simulink model "Copy_of_RoboCarModel"  (R2023a)
settings: Solver=VariableStepAuto  StartTime=0.0  StopTime=10.0  RelTol=1e-3
settings Model: Creator=Franz  LastModifiedBy=Franz

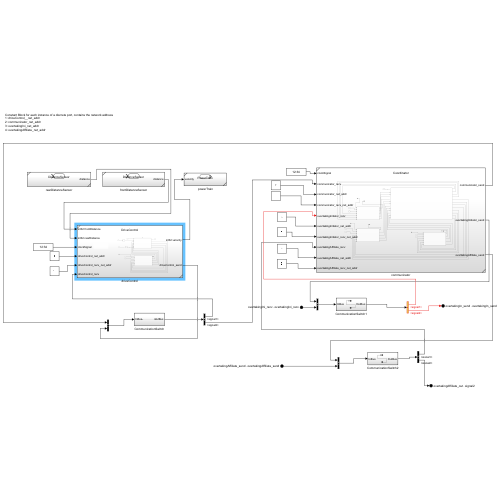
[thumbnail: Simulink's stored preview of the top-level diagram]
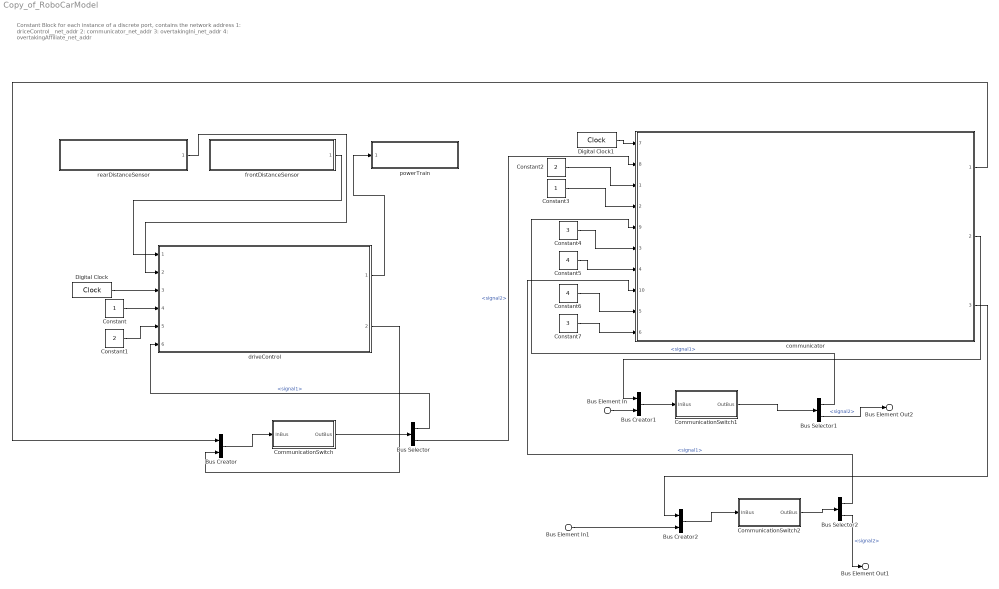
== system Copy_of_RoboCarModel ==
  note: Constant Block for each instance of a discrete port, contains the network address
      | 1: driceControl__net_addr
      | 2: communicator_net_addr
      | 3: overtakingIni_net_addr
      | 4: overtakingAffiliate_net_addr
  Bus Element In : Inport  PortName=overtakingIni_recv  Element=overtakingIni_recv
  Bus Element In1 : Inport  Port=2  PortName=overtakingAffiliate_send  Element=overtakingAffiliate_send
  " powerTrain" : Subsystem  ReferencedSubsystem=PowerTrain
  Bus Creator : BusCreator  Inputs=2
  Bus Creator1 : BusCreator  Inputs=2
  Bus Creator2 : BusCreator  Inputs=2
  Bus Selector : BusSelector  OutputSignals=signal1,signal2
  Bus Selector1 : BusSelector  OutputSignals=signal1,signal2
  Bus Selector2 : BusSelector  OutputSignals=signal1,signal2
  CommunicationSwitch : Subsystem
  CommunicationSwitch1 : Subsystem
  CommunicationSwitch2 : Subsystem
  Constant : Constant
  Constant1 : Constant  Value=2
  Constant2 : Constant  Value=2
  Constant3 : Constant
  Constant4 : Constant  Value=3
  Constant5 : Constant  Value=4
  Constant6 : Constant  Value=4
  Constant7 : Constant  Value=3
  Digital Clock : DigitalClock
  Digital Clock1 : DigitalClock
  communicator : Subsystem  ReferencedSubsystem=Coordinator
      settings: PortSchema="{\"entries\":[{\"content\":{\"sides\":[{\"content\":{\"connectorIds\":[\"In7\",\"In8\",\"In1\",\"In2\",\"In9\",\"In3\",\"In4\",\"In10\",\"In5\",\"In6\"]},\"type\":\"ConnectorPlacement.EquallySpacedRectSide\",\"uuid\":\"597f2600-0266-49ee-88a2-3e6a618a9f6e\"},{\"content\":{\"connectorIds\":[\"Out1\",\"Out2\",\"Out3\"],\"side\":\"RIGHT\"},\"type\":\"ConnectorPlacement.EquallySpacedRectSide\",\"uuid\":\"8a05e0df-8602-4cac-b3df-55f21ffd748f\"},{\"content\":{\"side\":\"TOP\"},\"type\":\"ConnectorPlacement.EquallySpacedRectSide\",\"uuid\":\"f3d30c22-937d-4096-90b7-da40b4c40188\"}]},\"type\":\"ConnectorPlacement.EquallySpacedConnector\",\"uuid\":\"be54317e-1502-459c-b560-7b4d203f7350\"}],\"packageUris\":[\"http://schema.mathworks.com/mf0/Connector/R2020b\"],\"version\":\"1.0\"}"
  driveControl : Subsystem  ReferencedSubsystem=DriveControl
  frontDistanceSensor : Subsystem  ReferencedSubsystem=DistanceSensor
  rearDistanceSensor : Subsystem  ReferencedSubsystem=DistanceSensor
  Bus Element Out1 : Outport  PortName=overtakingAffiliate_out  Element=signal2
  Bus Element Out2 : Outport  Port=2  PortName=overtakingIn_send  Element=overtakingIn_send
  wires:
  frontDistanceSensor/1 -> driveControl/1
  driveControl/1 -> " powerTrain"/1
  rearDistanceSensor/1 -> driveControl/2
  Digital Clock/1 -> driveControl/3
  Bus Creator/1 -> CommunicationSwitch/1(InBus)
  CommunicationSwitch/1(OutBus) -> Bus Selector/1
  Constant/1 -> driveControl/4
  Constant1/1 -> driveControl/5
  Constant2/1 -> communicator/1
  Constant3/1 -> communicator/2
  Bus Creator1/1 -> CommunicationSwitch1/1(InBus)
  CommunicationSwitch1/1(OutBus) -> Bus Selector1/1
  Bus Creator2/1 -> CommunicationSwitch2/1(InBus)
  CommunicationSwitch2/1(OutBus) -> Bus Selector2/1
  Bus Selector2/1 -> communicator/10  "<signal1>"
  Constant4/1 -> communicator/3
  Constant5/1 -> communicator/4
  Constant6/1 -> communicator/5
  Constant7/1 -> communicator/6
  Digital Clock1/1 -> communicator/7
  driveControl/2 -> Bus Creator/2
  Bus Selector/1 -> driveControl/6  "<signal1>"
  Bus Element In/1 -> Bus Creator1/2
  Bus Selector2/2 -> Bus Element Out1/1  "<signal2>"
  Bus Element In1/1 -> Bus Creator2/2
  Bus Selector/2 -> communicator/8  "<signal2>"
  communicator/1 -> Bus Creator/1
  communicator/3 -> Bus Creator2/1
  communicator/2 -> Bus Creator1/1
  Bus Selector1/2 -> Bus Element Out2/1  "<signal2>"
  Bus Selector1/1 -> communicator/9  "<signal1>"

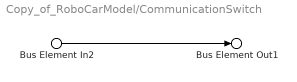
== system Copy_of_RoboCarModel/CommunicationSwitch ==
  Bus Element In2 : Inport  PortName=InBus  Element=signal1
  Bus Element Out1 : Outport  PortName=OutBus  Element=signal1
  wires:
  Bus Element In2/1 -> Bus Element Out1/1

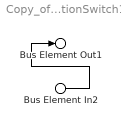
== system Copy_of_RoboCarModel/CommunicationSwitch1 ==
  Bus Element In2 : Inport  PortName=InBus  Element=signal1
  Bus Element Out1 : Outport  PortName=OutBus  Element=signal1
  wires:
  Bus Element In2/1 -> Bus Element Out1/1

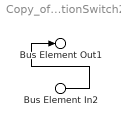
== system Copy_of_RoboCarModel/CommunicationSwitch2 ==
  Bus Element In2 : Inport  PortName=InBus  Element=signal1
  Bus Element Out1 : Outport  PortName=OutBus  Element=signal1
  wires:
  Bus Element In2/1 -> Bus Element Out1/1
